simulink model "Convert_meter_to_feet"  (R2022b)
settings: Solver=VariableStepAuto  StartTime=0.0  StopTime=10.0  RelTol=1e-3
settings Model: Creator=Dell  LastModifiedBy=Dell

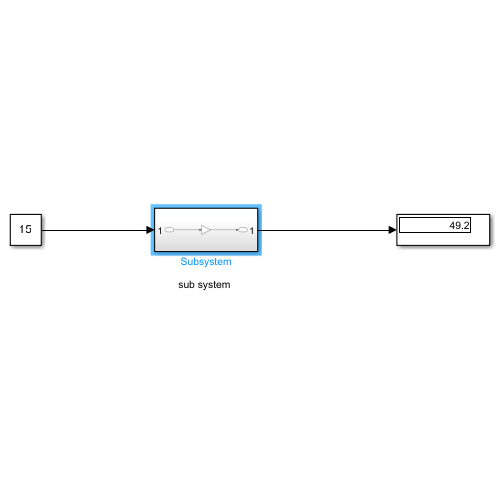
[thumbnail: Simulink's stored preview of the top-level diagram]
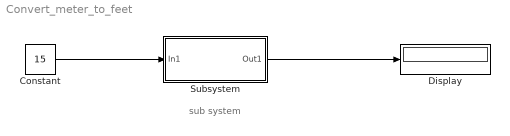
== system Convert_meter_to_feet ==
  note: sub system
  Constant : Constant  Value=15
  Display : Display
  Subsystem : Subsystem
  wires:
  Constant/1 -> Subsystem/1(In1)
  Subsystem/1(Out1) -> Display/1

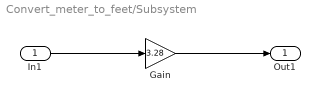
== system Convert_meter_to_feet/Subsystem ==
  In1 : Inport
  Gain : Gain  Gain=3.28
  Out1 : Outport
  wires:
  Gain/1 -> Out1/1
  In1/1 -> Gain/1
